simulink model "aula1_mma_2018"  (R2018a)
settings: Solver=VariableStepAuto  StartTime=0.0  StopTime=20  RelTol=1e-3
values from neighbouring files (symbols this model uses):
  k = z1(i)    [init.m]
  m = z2(i)    [init.m]
undefined symbols (not defined in the file or in its folder): b, F
settings Model: Creator=celsojosemunaro  LastModifiedBy=celsojosemunaro
settings DataIOCC: ReturnWorkspaceOutputs=on
settings SFSimCC: SimUseLocalCustomCode=on
settings RTWCC: RTWUseLocalCustomCode=on

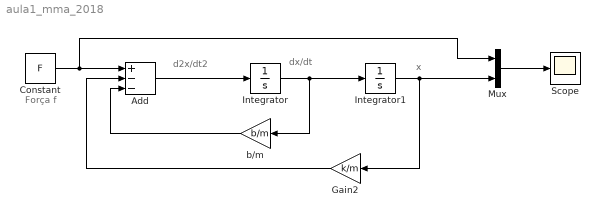
== system aula1_mma_2018 ==
  note: d2x/dt2
  note: dx/dt
  note: x
  note: Força f
  Add : Sum  Inputs=+--
  Constant : Constant  Value=F
  Gain2 : Gain  Gain=k/m
  Integrator : Integrator
  Integrator1 : Integrator
  Mux : Mux  Inputs=2
  Scope : Scope
  b/m : Gain  Gain=b/m
  wires:
  Constant/1 -> Mux/1, Add/1
  Add/1 -> Integrator/1
  Integrator/1 -> b/m/1, Integrator1/1
  b/m/1 -> Add/3
  Integrator1/1 -> Mux/2, Gain2/1
  Gain2/1 -> Add/2
  Mux/1 -> Scope/1
